simulink model "serial_variables_corrected"  (R2019a)
settings: Solver=VariableStepAuto  StartTime=0.0  StopTime=10.0  RelTol=1e-3
libraries: etargetslib x14, frdmk64flib x1
settings Model: Creator=Laura  LastModifiedBy=Laura

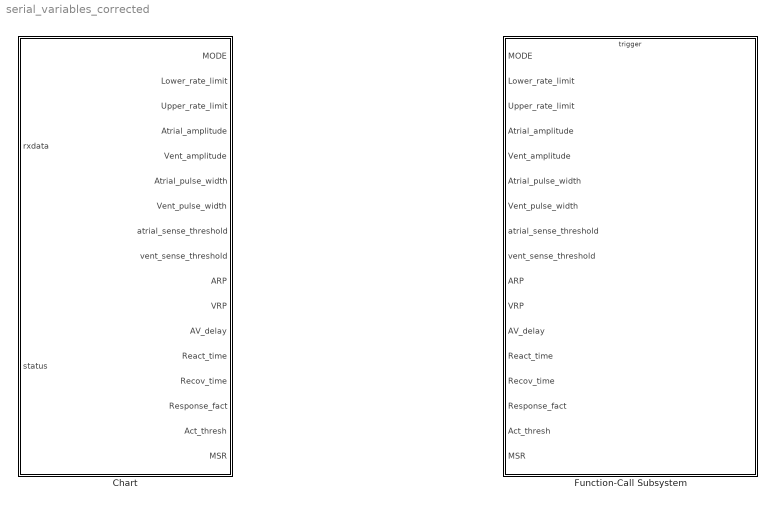
== system serial_variables_corrected ==
  Chart : Stateflow chart  BlockKeywords=__PRM__SERIALIZED__DATA__:Stateflow Chart,Stateflow Diagram  TreatAsAtomicUnit=on
  Function-Call Subsystem : Subsystem  TreatAsAtomicUnit=on

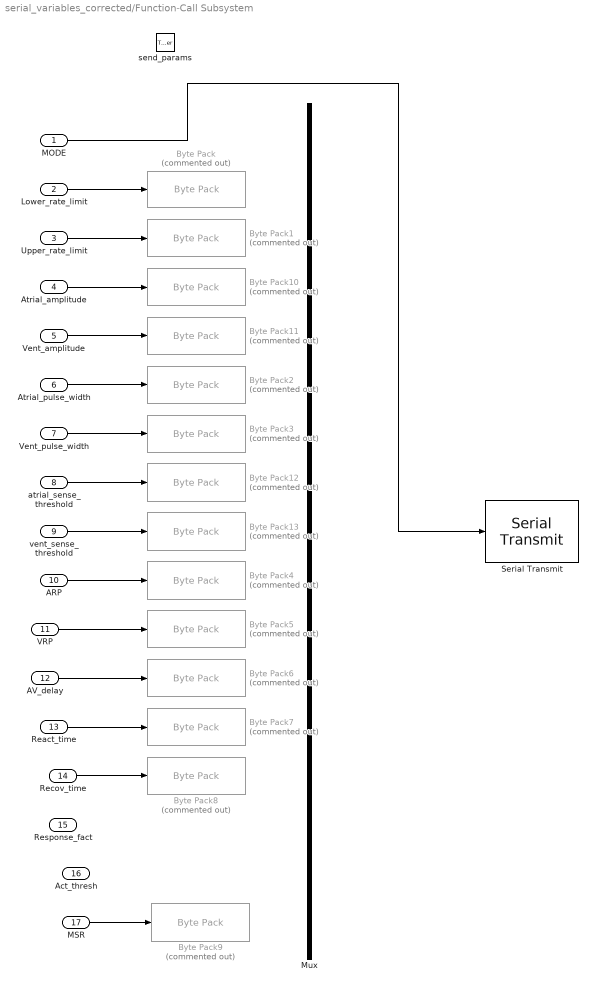
== system serial_variables_corrected/Function-Call Subsystem ==
  MODE : Inport
  Lower_rate_limit : Inport  Port=2
  Upper_rate_limit : Inport  Port=3
  Atrial_amplitude : Inport  Port=4
  Vent_amplitude : Inport  Port=5
  Atrial_pulse_width : Inport  Port=6
  Vent_pulse_width : Inport  Port=7
  atrial_sense_threshold : Inport  Port=8
  vent_sense_threshold : Inport  Port=9
  ARP : Inport  Port=10
  VRP : Inport  Port=11
  AV_delay : Inport  Port=12
  React_time : Inport  Port=13
  Recov_time : Inport  Port=14
  Response_fact : Inport  Port=15
  Act_thresh : Inport  Port=16
  MSR : Inport  Port=17
  send_params : TriggerPort  TriggerType=function-call  IsSimulinkFunction=on  FunctionName=send_params  VariantControl=Variant
  Byte Pack{,1..9} (10 alike) : etargetslib/Byte Pack  Commented=on  datatypes={'uint16'}  byteAlign=1
      settings: SourceProductName=MATLAB Coder
  Byte Pack{10..13} (4 alike) : etargetslib/Byte Pack  Commented=on  datatypes={'double'}  byteAlign=1
      settings: SourceProductName=MATLAB Coder
  Mux : Mux  Inputs=17
  Serial Transmit : frdmk64flib/Serial Transmit  SCIModule=0  Baudrate=uint32(9600)  Parity=None  StopBits=1  HardwareFlowControl=None  ByteOrder=LittleEndian  BlockingMode=on  OutputStatus=off
      settings: SourceProductName=Simulink Coder Support Package for NXP FRDM-K64F Board
  wires:
  MSR/1 -> Byte Pack9/1
  AV_delay/1 -> Byte Pack6/1
  VRP/1 -> Byte Pack5/1
  Recov_time/1 -> Byte Pack8/1
  vent_sense_threshold/1 -> Byte Pack13/1
  ARP/1 -> Byte Pack4/1
  Upper_rate_limit/1 -> Byte Pack1/1
  Vent_amplitude/1 -> Byte Pack11/1
  Atrial_amplitude/1 -> Byte Pack10/1
  React_time/1 -> Byte Pack7/1
  Atrial_pulse_width/1 -> Byte Pack2/1
  atrial_sense_threshold/1 -> Byte Pack12/1
  Lower_rate_limit/1 -> Byte Pack/1
  Vent_pulse_width/1 -> Byte Pack3/1
  MODE/1 -> Serial Transmit/1

== stateflow chart serial_variables_corrected/Chart ==
  state SET_PARAMS
    %we assume this is the order that the data is sent in
    entry:
    %MODE = rxdata(1);
    %Lower_rate_limit = typecast(rxdata(2:3), 'uint16');
    %Upper_rate_limit = typecast(rxdata(4:5), 'uint16');
    %Atrial_amplitude = typecast(rxdata(6:13), 'double');
    %Vent_amplitude = typecast(rxdata(14:21), 'double');
    %Atrial_pulse_width = typecast(rxdata(22:23), 'uint16');
    %Vent_pulse_width = typecast(rxdata(24:25), 'uint16')
    %atrial_sense_threshold = typecast(rxdata(26:33), 'double')
    %vent_sense_threshold = typecast(rxdata(34:41), 'double')
    %ARP = typecast(rxdata(42:43), 'uint16')
    %VRP = typecast(rxdata(44:45), 'uint16')
    %AV_delay = typecast(rxdata(46:47), 'uint16')
    %React_time = typecast(rxdata(48:49), 'uint16')
    %Recov_time = typecast(rxdata(50:51), 'uint16')
    %Response_fact = rxdata(52)
    %Act_thresh = rxdata(53)
    %MSR = typecast(rxdata(54:55), 'uint16')
    send_params();
  state INITIAL
    entry:
    MODE = 1;
    Lower_rate_limit = 60;
    Upper_rate_limit = 120;
    Atrial_amplitude = 3.3;
    Vent_amplitude = 3.3;
    Atrial_pulse_width = 10;
    Vent_pulse_width = 10;
    atrial_sense_threshold = 2.75;
    vent_sense_threshold = 2.75;
    ARP = 300;
    VRP = 300;
    AV_delay = 100;
    React_time = 0; %unknown
    Recov_time = 0; %unknown
    Response_fact = 0; %unknown
    Act_thres = 0; %unknown
    MSR = 0; %unknown
  state STANDBY
    %Waiting for COM
  note: status == 0 indicates successful read
  (default) -> INITIAL
  SET_PARAMS -> STANDBY
  STANDBY -> SET_PARAMS : [status == 0]
  INITIAL -> STANDBY
  data: rxdata input uint8; status input uint8; MODE output uint8; Lower_rate_limit output uint16; Upper_rate_limit output uint16; Atrial_amplitude output double; Vent_amplitude output double; Atrial_pulse_width output uint16; Vent_pulse_width output uint16; atrial_sense_threshold output double; vent_sense_threshold output double; ARP output uint16; VRP output uint16; AV_delay output uint16; React_time output uint16; Recov_time output uint16; Response_fact output uint8; Act_thresh output uint8; MSR output uint16
